simulink library "eq_lib"  (Simulink 6.0)
settings: Solver=ode45  SolverMode=SingleTasking  StartTime=0.0  StopTime=10.0  RelTol=1e-3
undefined symbols (not defined in the file or in its folder): qammod
libraries: commeq2 x7
settings Model: Creator=arodrigu  LastModifiedBy=arodrigu
settings DataIOCC: SignalLoggingName=logsOut
settings OptimizationCC: BooleanDataType=off
settings DebuggingCC: CheckExecutionContextPreStartOutputMsg=on  CheckExecutionContextRuntimeOutputMsg=on  SolverPrmCheckMsg=none
settings HardwareCC: TargetUnknown=on
settings ModelReferenceCC: UpdateModelReferenceTargets=IfOutOfDate
settings GRTTargetCC: LifeSpan=inf
settings SFSimCC: SFSimApplyToAllLibs=on  SFSimBuildMode=Incremental

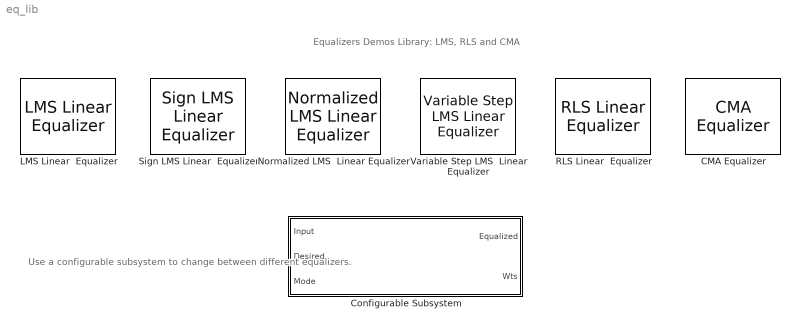
== system eq_lib ==
  note: Equalizers Demos Library: LMS, RLS and CMA
  note: Use a configurable
      | subsystem to change between
      | different equalizers.
  CMA Equalizer : commeq2/CMA Equalizer  nTaps=4  nSamp=1  sigConst=qammod([0:15],16)  stepSize=0.01  leakage=1  initWeights=0  outErr=off  outWeights=on
  Configurable Subsystem : Subsystem  BlockChoice="LMS Linear  Equalizer"  EnableExecutionContextPropagation=on
      settings: TemplateBlock=self  MemberBlocks="CMA Equalizer,LMS Linear  Equalizer,Normalized LMS  Linear Equalizer,RLS Linear  Equalizer,Sign LMS Linear  Equalizer,Variable Step LMS  Linear Equalizer"
      mask Display: disp(get_param(gcb,'BlockChoice'))
  LMS Linear  Equalizer : commeq2/LMS Linear  Equalizer  nTaps=4  nSamp=1  sigConst=qammod([0:15],16)  delay=2  stepSize=0.01  leakage=1  initWeights=0  mode=on  outErr=off  outWeights=on
  Normalized LMS  Linear Equalizer : commeq2/Normalized LMS  Linear Equalizer  nTaps=4  nSamp=1  sigConst=qammod([0:15],16)  delay=2  stepSize=0.01  leakage=1  bias=1  initWeights=0  mode=on  outErr=off  outWeights=on
  RLS Linear  Equalizer : commeq2/RLS Linear  Equalizer  nTaps=4  nSamp=1  sigConst=qammod([0:15],16)  delay=2  lambda=.99  invCorr=.1*eye(4)  initWeights=0  mode=on  outErr=off  outWeights=on
  Sign LMS Linear  Equalizer : commeq2/Sign LMS Linear  Equalizer  alg=Sign LMS  nTaps=4  nSamp=1  sigConst=qammod([0:15],16)  delay=2  stepSize=0.01  leakage=1  initWeights=0  mode=on  outErr=off  outWeights=on
  Variable Step LMS  Linear Equalizer : commeq2/Variable Step LMS  Linear Equalizer  nTaps=4  nSamp=1  sigConst=qammod([0:15],16)  delay=2  initMu=.01  incMu=.01  minMu=.001  maxMu=.1  leakage=1  initWeights=0  mode=on  outErr=off  outWeights=on

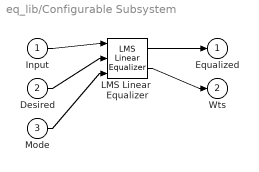
== system eq_lib/Configurable Subsystem ==
  Input : Inport  LatchInput=off
  Desired : Inport  Port=2  LatchInput=off
  Mode : Inport  Port=3  LatchInput=off
  LMS Linear  Equalizer : commeq2/LMS Linear  Equalizer  nTaps=4  nSamp=1  sigConst=qammod([0:15],16)  delay=2  stepSize=0.01  leakage=1  initWeights=0  mode=on  outErr=off  outWeights=on
  Equalized : Outport
  Wts : Outport  Port=2
  wires:
  Input/1 -> LMS Linear  Equalizer/1
  Desired/1 -> LMS Linear  Equalizer/2
  Mode/1 -> LMS Linear  Equalizer/3
  LMS Linear  Equalizer/1 -> Equalized/1
  LMS Linear  Equalizer/2 -> Wts/1
